simulink model "tut2_3"  (R2019b)
settings: Solver=VariableStepAuto  StartTime=0.0  StopTime=simTime  RelTol=1e-3
values from neighbouring files (symbols this model uses):
  di_fv = 0.5    [tut2.m]
  di_step = 50    [tut2.m]
  do_fv = 0.5    [tut2.m]
  do_step = 100    [tut2.m]
libraries: cstblocks x8
settings Model: Creator=c3277928  LastModifiedBy=c3277928

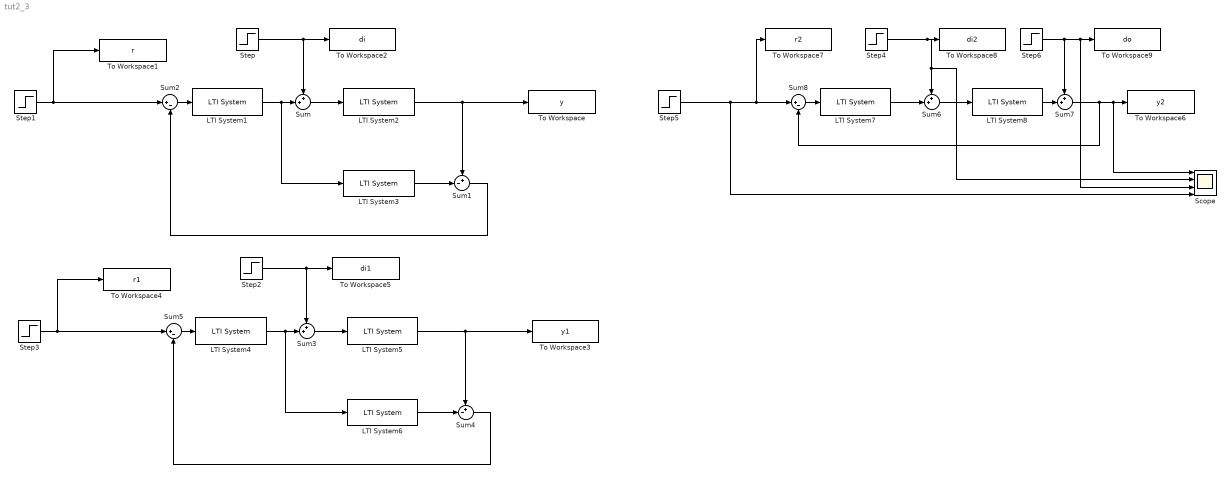
== system tut2_3 ==
  LTI System1 : cstblocks/LTI System  sys=Q  IC=[]
  LTI System2 : cstblocks/LTI System  sys=G  IC=[]
  LTI System3 : cstblocks/LTI System  sys=G0  IC=[]
  LTI System4 : cstblocks/LTI System  sys=Q1  IC=[]
  LTI System5 : cstblocks/LTI System  sys=G  IC=[]
  LTI System6 : cstblocks/LTI System  sys=G0  IC=[]
  LTI System7 : cstblocks/LTI System  sys=C  IC=[]
  LTI System8 : cstblocks/LTI System  sys=G  IC=[]
  Scope : Scope  NumInputPorts=4
  Step : Step  Time=di_step  After=di_fv  SampleTime=0
  Step1 : Step  SampleTime=0
  Step2 : Step  Time=di_step  After=di_fv  SampleTime=0
  Step3 : Step  SampleTime=0
  Step4 : Step  Time=di_step  After=di_fv  SampleTime=0
  Step5 : Step  SampleTime=0
  Step6 : Step  Time=do_step  After=do_fv  SampleTime=0
  Sum{,3,6..7} (4 alike) : Sum  Inputs=++|
  Sum1 : Sum  Inputs=+-|
  Sum2 : Sum  Inputs=|+-
  Sum4 : Sum  Inputs=+-|
  Sum5 : Sum  Inputs=|+-
  Sum8 : Sum  Inputs=|+-
  To Workspace : ToWorkspace  VariableName=y  SaveFormat=Timeseries  SampleTime=-1
  To Workspace1 : ToWorkspace  VariableName=r  SaveFormat=Timeseries  SampleTime=-1
  To Workspace2 : ToWorkspace  VariableName=di  SaveFormat=Timeseries  SampleTime=-1
  To Workspace3 : ToWorkspace  VariableName=y1  SaveFormat=Timeseries  SampleTime=-1
  To Workspace4 : ToWorkspace  VariableName=r1  SaveFormat=Timeseries  SampleTime=-1
  To Workspace5 : ToWorkspace  VariableName=di1  SaveFormat=Timeseries  SampleTime=-1
  To Workspace6 : ToWorkspace  VariableName=y2  SaveFormat=Timeseries  SampleTime=-1
  To Workspace7 : ToWorkspace  VariableName=r2  SaveFormat=Timeseries  SampleTime=-1
  To Workspace8 : ToWorkspace  VariableName=di2  SaveFormat=Timeseries  SampleTime=-1
  To Workspace9 : ToWorkspace  VariableName=do  SaveFormat=Timeseries  SampleTime=-1
  wires:
  Sum2/1 -> LTI System1/1
  Step/1 -> To Workspace2/1, Sum/1
  Sum/1 -> LTI System2/1
  Step1/1 -> Sum2/1, To Workspace1/1
  LTI System1/1 -> LTI System3/1, Sum/2
  Sum1/1 -> Sum2/2
  LTI System3/1 -> Sum1/2
  LTI System2/1 -> To Workspace/1, Sum1/1
  LTI System6/1 -> Sum4/2
  LTI System5/1 -> To Workspace3/1, Sum4/1
  Step3/1 -> Sum5/1, To Workspace4/1
  LTI System4/1 -> LTI System6/1, Sum3/2
  Sum3/1 -> LTI System5/1
  Sum5/1 -> LTI System4/1
  Step2/1 -> To Workspace5/1, Sum3/1
  Sum4/1 -> Sum5/2
  Sum6/1 -> LTI System8/1
  Step5/1 -> Scope/4, To Workspace7/1, Sum8/1
  LTI System7/1 -> Sum6/2
  Step4/1 -> Scope/2, Sum6/1, To Workspace8/1
  Sum8/1 -> LTI System7/1
  LTI System8/1 -> Sum7/2
  Sum7/1 -> Sum8/2, Scope/1, To Workspace6/1
  Step6/1 -> Scope/3, To Workspace9/1, Sum7/1
